simulink model "Z_AlgebraicLoops"  (R2017b)
settings: Solver=ode45  StartTime=0.0  StopTime=1  FixedStep=0.0005  MaxStep=1e-4  RelTol=1e-3  EnableMultiTasking=on
model workspace (MAT data in the model file):
  C = 0.001
  R = 1000
  Ri = 1000
settings Model: Creator=jbaur  LastModifiedBy=jbaur
settings DataIOCC: SaveFormat=StructureWithTime
settings OptimizationCC: ExpressionDepthLimit=2147483647  LifeSpan=inf
settings DebuggingCC: SolverPrmCheckMsg=warning  StateNameClashWarn=warning  SFUnexpectedBacktrackingDiag=warning  SFNoUnconditionalDefaultTransitionDiag=warning  SFExecutionAtInitializationDiag=none
settings HardwareCC: ProdBitPerInt=16  ProdBitPerPointer=8  ProdBitPerSizeT=16  ProdBitPerPtrDiffT=16  ProdLargestAtomicFloat=None  ProdEndianess=Unspecified  ProdWordSize=8  ProdShiftRightIntArith=off  ProdHWDeviceType=Intel->8051 Compatible
settings ModelReferenceCC: PropagateSignalLabelsOutOfModel=off
settings RTWCC: GenerateReport=on  LaunchReport=on
settings CodeAppCC: StateflowObjectComments=on
settings GRTTargetCC: TargetLangStandard=C89/C90 (ANSI)  GeneratePreprocessorConditionals=Disable all  CombineOutputUpdateFcns=off  GRTInterface=on
settings ConfigComp: CovMetricSettings=dw  CovHtmlReporting=on  CovSaveCumulativeToWorkspaceVar=on  CovSaveSingleToWorkspaceVar=on  CovExternalEMLEnable=off  CovSFcnEnable=off

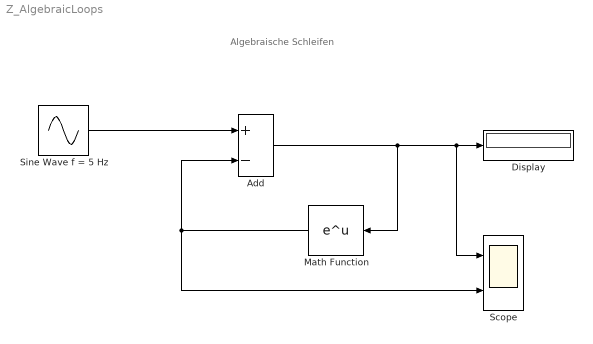
== system Z_AlgebraicLoops ==
  note: Algebraische Schleifen
  Add : Sum  Inputs=+-
  Display : Display
  Math Function : Math  SaturateOnIntegerOverflow=on
  Scope : Scope  NumInputPorts=2
  Sine Wave f = 5 Hz : Sin  Frequency=2*pi*5  SampleTime=0
  wires:
  Sine Wave f = 5 Hz/1 -> Add/1
  Add/1 -> Display/1, Scope/1, Math Function/1
  Math Function/1 -> Add/2, Scope/2
